simulink model "kalman_estimate_MM"  (R2018b)
settings: Solver=FixedStepAuto  StartTime=0.0  StopTime=500  FixedStep=0.02  RelTol=1e-3
values from neighbouring files (symbols this model uses):
  D = randn(num_output,num_control)    [Com_of_linear_model_calculate.m]    (also in Copy_of_linear_model_calculate.m; D.mat = [0 0 0.00507528406191 0.0236369284061 0.221173094143 0.00198; LINEAR.m = randn(8,1)*10; MM_HKF.m = reshape(out(A_l+B_l+C_l+1:A_l+B_l+C_l+D_l),size_D))
undefined symbols (not defined in the file or in its folder): act_piece, com_piece, piece, sigbuilder_block
libraries: sharedschedule x467, dspsigattribs x44, commchan3 x1
(part 1 of 5)
settings Model: Creator=mmm  LastModifiedBy=mmm

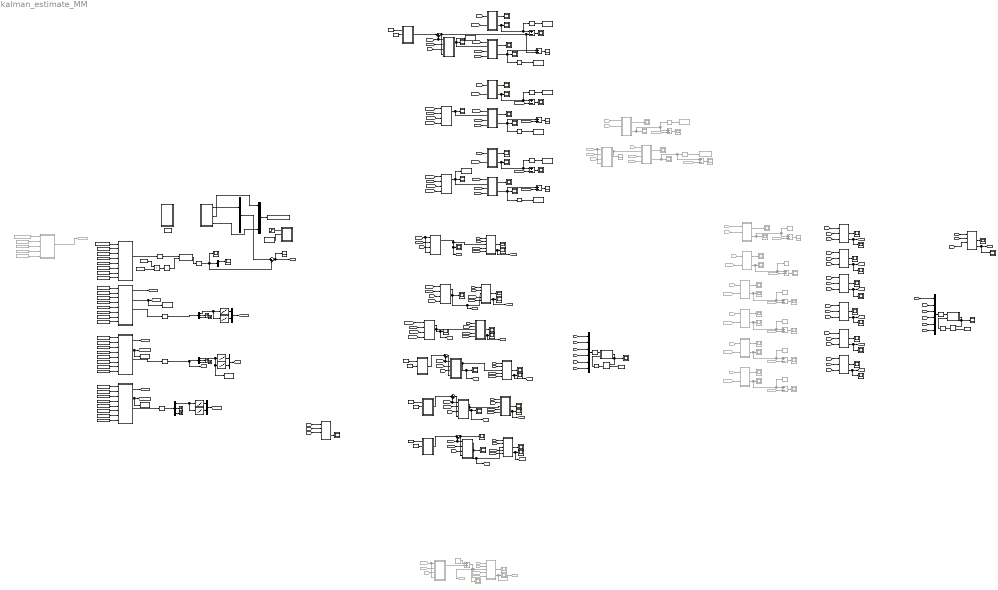
== system kalman_estimate_MM ==
  note: fHPT decrease 3 percent a7
  note: actuator fault a2
  note: T3 fault a5
  note: P21 fault a4
  note: Nh fault a3
  note: boost fault a2
  note: no fault a1
  note: 无故障模式下模型对比
  note: 增压级故障模型对比
  note: 执行机构故障模型对比
  note: 增压级故障模型对比
  1-D Lookup Table1 : Lookup_n-D  NumberOfTableDimensions=1  BreakpointsForDimension1=com_piece.u_stable_(:,1)  Table=com_piece.Nl  InterpMethod=Cubic spline  ExtrapMethod=Cubic spline  InternalRulePriority=Speed  RndMeth=Simplest  InputSameDT=on
  1-D Lookup Table2 : Lookup_n-D  NumberOfTableDimensions=1  BreakpointsForDimension1=piece.u_stable_(:,1)  Table=piece.Nl  InterpMethod=Cubic spline  ExtrapMethod=Cubic spline  InternalRulePriority=Speed  RndMeth=Simplest  InputSameDT=on
  1-D Lookup Table3 : Lookup_n-D  NumberOfTableDimensions=1  BreakpointsForDimension1=piece.u_stable_(:,1)  Table=piece.x_stable_(:,2)  InterpMethod=Cubic spline  ExtrapMethod=Cubic spline  InternalRulePriority=Speed  RndMeth=Simplest  InputSameDT=on
  1-D Lookup Table4 : Lookup_n-D  NumberOfTableDimensions=1  BreakpointsForDimension1=com_piece.u_stable_(:,1)  Table=com_piece.x_stable_(:,2)  InterpMethod=Cubic spline  ExtrapMethod=Cubic spline  InternalRulePriority=Speed  RndMeth=Simplest  InputSameDT=on
  1-D Lookup Table5 : Lookup_n-D  NumberOfTableDimensions=1  BreakpointsForDimension1=act_piece.u_stable_(:,1)  Table=act_piece.Nl  InterpMethod=Cubic spline  ExtrapMethod=Cubic spline  InternalRulePriority=Speed  RndMeth=Simplest  InputSameDT=on
  1-D Lookup Table6 : Lookup_n-D  NumberOfTableDimensions=1  BreakpointsForDimension1=act_piece.u_stable_(:,1)  Table=act_piece.x_stable_(:,2)  InterpMethod=Cubic spline  ExtrapMethod=Cubic spline  InternalRulePriority=Speed  RndMeth=Simplest  InputSameDT=on
  AKF1 : Subsystem
  AKF10 : Subsystem  Commented=on
  AKF12 : Subsystem
  AKF2 : Subsystem
  AKF3 : Subsystem
  AKF4 : Subsystem
  AKF5 : Subsystem
  AKF6 : Subsystem
  AKF7 : Subsystem  Commented=on
  AKF8 : Subsystem
  AKF9 : Subsystem
  AWGN Channel1 : commchan3/AWGN Channel  InputProcessing=Columns as channels (frame based)  seed=51:60  noiseMode=Variance from port  EbNodB=10  EsNodB=10  SNRdB=10  bitsPerSym=1  Ps=1  Tsym=1  variance=[2.55,7.5,0.03,0.03,0.3,0.3,0.15,0.15,0.45,0.45].^2
  Add1 : Sum  Commented=on
  Constant : Constant  Commented=on  Value=[0,0,0,0,0,0,0,0,-0.03,0]  VectorParams1D=off
  Constant{1,4,8,23} (4 alike) : Constant  Value=piece.Ny(:,:,1)
  Constant{10,19,22,24} (4 alike) : Constant  Value=piece.y_index
  Constant{11,25,30,35} (4 alike) : Constant  Value=piece.U_index
  Constant{12,26,31,36} (4 alike) : Constant  Value=piece.x_index
  Constant13 : Constant  Value=[0.051,0.051,0.164,0.164,0.15,0.15,0.23,0.23,0.097,0.097]  VectorParams1D=off
  Constant14 : Constant  Value=0.01
  Constant15 : Constant  Commented=on  Value=piece.HP_index
  Constant16 : Constant  Commented=on  Value=piece.y_index
  Constant17 : Constant  Commented=on  Value=piece.U_index
  Constant18 : Constant  Commented=on  Value=piece.x_index
  Constant{2,27,32,37} (4 alike) : Constant  Value=piece.Nu(:,:,1)
  Constant20 : Constant  Commented=on  Value=piece.mean_design  VectorParams1D=off
  Constant21 : Constant  Value=[0.9,0.01,0.01,0.01,0.01,0.01]  VectorParams1D=off
  Constant{3,28,33,38} (4 alike) : Constant  Value=piece.Nx(:,:,1)
  Constant{9,29,34,39} (4 alike) : Constant  Value=piece.HP_index
  Constant40 : Constant  Value=0
  Constant41 : Constant  Value=[0.9,0.01,0.01,0.01,0.01,0.01]  VectorParams1D=off
  Constant{5..7,42} (4 alike) : Constant  Value=-0.03
  Delay : Delay  DelayLength=1  InitialConditionSource=Input port
      settings: InputPortMap=u0,p4
  Delay1 : Delay  DelayLength=1  InitialConditionSource=Input port
      settings: InputPortMap=u0,p4
  Demux1 : Demux  Outputs=3
  Demux2 : Demux  Outputs=3
  Demux4 : Demux  Outputs=3
  Demux5 : Demux  Outputs=[1,9]
  From{53,71,79,89,92,95,100} (7 alike) : From  Commented=on  GotoTag=y_obem
  From{14,27,39,42,57} (5 alike) : From  Commented=on  GotoTag=y_obem1
  From{21,28,40,47,76} (5 alike) : From  Commented=on  GotoTag=com_x0
  From{26,29,41,46,52,96..97} (7 alike) : From  Commented=on  GotoTag=u
  From{54,69,90..91} (4 alike) : From  Commented=on  GotoTag=x_obem
  From{55..56,72,93..94,99} (6 alike) : From  Commented=on  GotoTag=x0
  From70 : From  Commented=on  GotoTag=y
  Goto31 : Goto  Commented=on  GotoTag=H7
  Goto5 : Goto  Commented=on  GotoTag=y_design
  Goto8 : Goto  Commented=on  GotoTag=f7
  HKF1 : Subsystem
  HKF10 : Subsystem
  HKF11 : Subsystem  Commented=on
  HKF2 : Subsystem
  HKF3 : Subsystem
  HKF4 : Subsystem
  HKF5 : Subsystem
  HKF6 : Subsystem
  HKF7 : Subsystem  Commented=on
  HKF8 : Subsystem
  HKF9 : Subsystem
  MATLAB Function : MATLAB Function  TreatAsAtomicUnit=on
  MATLAB Function1 : MATLAB Function  TreatAsAtomicUnit=on
  MATLAB Function2 : MATLAB Function  TreatAsAtomicUnit=on
  MATLAB Function3 : MATLAB Function  TreatAsAtomicUnit=on
  MATLAB Function4 : MATLAB Function  TreatAsAtomicUnit=on
  MATLAB Function5 : MATLAB Function  TreatAsAtomicUnit=on
  MATLAB Function8 : MATLAB Function  TreatAsAtomicUnit=on
  Math Function : Math  Operator=square  SaturateOnIntegerOverflow=on
  Minus{,3,10..13} (6 alike) : Sum  Inputs=+-
  Minus{1..2,4..9} (8 alike) : Sum  Commented=on  Inputs=+-
  Multiply : Product
  Mux : Mux  Inputs=6
  Mux1 : Mux  Inputs=6
  Mux2 : Mux  Inputs=10
  Mux3 : Mux  Inputs=2
  Mux4 : Mux  Inputs=6
  Mux5 : Mux  Inputs=2
  Mux6 : Mux  Inputs=2
  PIECE kalman : Subsystem
  PIECE kalman1 : Subsystem
  PWL : Subsystem  Commented=on
  Reshape{,4..5,8..9,15..16,19..22} (11 alike) : Reshape  OutputDimensionality=Row vector (2-D)
  Reshape{1,6..7,10..14} (8 alike) : Reshape  Commented=on  OutputDimensionality=Row vector (2-D)
  Reshape{2..3,17..18} (4 alike) : Reshape  OutputDimensionality=Column vector (2-D)
  Scope{1..3,5..6,8..14,16..17,19..21,23..24,26..27,30..32,34..36,38..41,60..88} (60 alike) : Scope
  Scope{4,7,15,18,22,25,28..29,33,37,42..59} (28 alike) : Scope  Commented=on
  Signal Builder : Subsystem  Tag=STV Subsys  LoadFcn=sigbuilder_block('load');  StartFcn=sigbuilder_block('start');  StopFcn=sigbuilder_block('stop');  ClipboardFcn=sigbuilder_block('clipboard');  mask(Sigbuilder block){tuvar=[0:10]}
      mask help: Simulink:masks:SigbuilderBlock_MD
      mask init:
      | if ~strcmp(get_param(bdroot(gcbh),'SimulationStatus'),'stopped') tuvar = sigbuilder_block('maskInit'); end
      settings: CopyFcn=sigbuilder_block('copy');  DeleteFcn=sigbuilder_block('delete');  ModelCloseFcn=sigbuilder_block('modelClose');  PreSaveFcn=sigbuilder_block('preSave');  PauseFcn=sigbuilder_block('pause');  ContinueFcn=sigbuilder_block('continue');  NameChangeFcn=sigbuilder_block('namechange');  OpenFcn=sigbuilder_block('open',[6 30 1428 681 ]);  CloseFcn=sigbuilder_block('close');
      mask Display: plot(0, 0, 100, 100,[2, 2, 32, 32, 2], [68, 8, 8, 68, 68],[32, 2], [38, 38], [32, 19, 2],[53, 60, 44], [32, 17, 17, 2],[16, 16, 31, 31]);txt = getActiveGroup(gcbh);text(2, 100, txt,'verticalAlignment', 'top');
  Signal Builder1 : Subsystem  Tag=STV Subsys  LoadFcn=sigbuilder_block('load');  StartFcn=sigbuilder_block('start');  StopFcn=sigbuilder_block('stop');  ClipboardFcn=sigbuilder_block('clipboard');  mask(Sigbuilder block){tuvar=[0:10]}
      mask help: Simulink:masks:SigbuilderBlock_MD
      mask init:
      | if ~strcmp(get_param(bdroot(gcbh),'SimulationStatus'),'stopped') tuvar = sigbuilder_block('maskInit'); end
      settings: CopyFcn=sigbuilder_block('copy');  DeleteFcn=sigbuilder_block('delete');  ModelCloseFcn=sigbuilder_block('modelClose');  PreSaveFcn=sigbuilder_block('preSave');  PauseFcn=sigbuilder_block('pause');  ContinueFcn=sigbuilder_block('continue');  NameChangeFcn=sigbuilder_block('namechange');  OpenFcn=sigbuilder_block('open',[6 30 1428 681 ]);  CloseFcn=sigbuilder_block('close');
      mask Display: plot(0, 0, 100, 100,[2, 2, 32, 32, 2], [68, 8, 8, 68, 68],[32, 2], [38, 38], [32, 19, 2],[53, 60, 44], [32, 17, 17, 2],[16, 16, 31, 31]);txt = getActiveGroup(gcbh);text(2, 100, txt,'verticalAlignment', 'top');
  Step : Step  Time=100  After=-0.08  SampleTime=0
  Sum{1..5} (5 alike) : Sum  Inputs=|++
  Terminator{1..6} (6 alike) : Terminator
  To Workspace : ToWorkspace  VariableName=fault_vector2  SampleTime=-1
      settings: Save2DSignal=2-D array (concatenate along first dimension)
  To Workspace1 : ToWorkspace  VariableName=y_obem2  SampleTime=-1
      settings: Save2DSignal=2-D array (concatenate along first dimension)
  To Workspace10 : ToWorkspace  VariableName=act_PWL  SampleTime=-1
      settings: Save2DSignal=2-D array (concatenate along first dimension)
  To Workspace11 : ToWorkspace  VariableName=sen3_HP_HKF  SampleTime=-1
      settings: Save2DSignal=2-D array (concatenate along first dimension)
  To Workspace12 : ToWorkspace  VariableName=sen3_PWL  SampleTime=-1
      settings: Save2DSignal=2-D array (concatenate along first dimension)
  To Workspace13 : ToWorkspace  VariableName=act_hp  SampleTime=-1
      settings: Save2DSignal=2-D array (concatenate along first dimension)
  To Workspace14 : ToWorkspace  VariableName=sen3_hp  SampleTime=-1
      settings: Save2DSignal=2-D array (concatenate along first dimension)
  To Workspace2 : ToWorkspace  VariableName=com_HP_HKF  SampleTime=-1
      settings: Save2DSignal=2-D array (concatenate along first dimension)
  To Workspace3 : ToWorkspace  VariableName=u  SaveFormat=Timeseries  SampleTime=-1
  To Workspace4 : ToWorkspace  VariableName=y_obem1  SampleTime=-1
      settings: Save2DSignal=2-D array (concatenate along first dimension)
  To Workspace5 : ToWorkspace  VariableName=com_PWL  SampleTime=-1
      settings: Save2DSignal=2-D array (concatenate along first dimension)
  To Workspace6 : ToWorkspace  Commented=on  VariableName=norm_PWL  SampleTime=-1
      settings: Save2DSignal=2-D array (concatenate along first dimension)
  To Workspace7 : ToWorkspace  Commented=on  VariableName=norm_HP_HKF  SampleTime=-1
      settings: Save2DSignal=2-D array (concatenate along first dimension)
  To Workspace8 : ToWorkspace  VariableName=y_obem  SampleTime=-1
      settings: Save2DSignal=2-D array (concatenate along first dimension)
  To Workspace9 : ToWorkspace  VariableName=act_HP_HKF  SampleTime=-1
      settings: Save2DSignal=2-D array (concatenate along first dimension)
  U1 : FromWorkspace  VariableName=model_test_com  SampleTime=0.02  Interpolate=off  OutputAfterFinalValue=Holding final value
  U2 : FromWorkspace  VariableName=model_test_health  SampleTime=0.02  Interpolate=off  OutputAfterFinalValue=Holding final value
  U3 : FromWorkspace  VariableName=model_test_act  SampleTime=0.02  Interpolate=off  OutputAfterFinalValue=Holding final value
  U4 : FromWorkspace  VariableName=model_test_health  SampleTime=0.02  Interpolate=off  OutputAfterFinalValue=Holding final value
  act_PIECE kalman : Subsystem
  act_PWL : Subsystem  Commented=on
  act_PWL_model : Subsystem
  com_PIECE kalman : Subsystem
  component_PWL : Subsystem  Commented=on
  component_PWL1 : Subsystem
  data_pre : MATLAB Function  TreatAsAtomicUnit=on
  data_pre1 : MATLAB Function  Commented=on  TreatAsAtomicUnit=on
  data_pre2 : MATLAB Function  TreatAsAtomicUnit=on
  data_pre3 : MATLAB Function  TreatAsAtomicUnit=on
  health_PWL : Subsystem  Commented=on
  no. of fault sensor : Constant  Value=8
  no. of fault sensor1 : Constant  Value=3
  no. of fault sensor3 : Constant  Value=2
  no. of fault sensor4 : Constant  Value=3
  no. of fault sensor5 : Constant  Value=8
  real_engine : MATLAB Function  TreatAsAtomicUnit=on
  sen2_PIECE kalman2 : Subsystem
  sen2_PWL : Subsystem  Commented=on
  sen3_PIECE kalman1 : Subsystem
  sen3_PIECE kalman3 : Subsystem
  sen3_PWL : Subsystem  Commented=on
  sen3_PWL-model : Subsystem
  sen8_PIECE kalman : Subsystem
  sen8_PWL : Subsystem  Commented=on
  wires:
  Reshape2/1 -> Demux4/1, [u]
  Demux4/1 -> To Workspace3/1, 1-D Lookup Table3/1, 1-D Lookup Table2/1
  Constant18/1 -> data_pre1/5(x_index)
  Reshape3/1 -> Sum2/2, Demux5/1, Scope10/1
  Constant9/1 -> data_pre/3(HP_index)
  Demux5/1 -> Scope9/1
  data_pre/2(y) -> To Workspace4/1, [y_obem1]
  Reshape/1 -> AWGN Channel1/1
  data_pre1/2(y) -> Goto5/1
  Constant16/1 -> data_pre1/2(y_index)
  Constant17/1 -> data_pre1/4(U_index)
  Constant15/1 -> data_pre1/3(HP_index)
  Constant12/1 -> data_pre/5(x_index)
  Constant11/1 -> data_pre/4(U_index)
  U1/1 -> data_pre/1(row_data)
  1-D Lookup Table2/1 -> Mux5/1
  no. of fault sensor/1 -> MATLAB Function/2(no)
  Constant10/1 -> data_pre/2(y_index)
  Mux5/1 -> [x0]
  1-D Lookup Table3/1 -> Mux5/2
  Constant13/1 -> Multiply/1
  Constant14/1 -> Multiply/2
  AWGN Channel1/1 -> Reshape3/1
  Sum2/1 -> Scope5/1, [y]
  Demux4/3 -> Terminator4/1
  Constant20/1 -> data_pre1/1(row_data)
  Math Function/1 -> AWGN Channel1/2
  Demux4/2 -> Terminator3/1
  Multiply/1 -> Math Function/1
  Constant2/1 -> data_pre/8(Nu)
  Constant1/1 -> data_pre/7(Ny)
  Constant3/1 -> data_pre/6(Nx)
  PIECE kalman/2(Out2) -> Scope12/1
  [u] -> PIECE kalman/1(In1)
  [x0] -> PIECE kalman/3(In3)
  [y] -> PIECE kalman/2(In2)
  data_pre/1(x) -> [x_obem1]
  [y_obem] -> HKF1/5(y_obem)
  [x_obem] -> HKF1/4(x_obem)
  HKF1/2(Out2) -> Scope13/1
  [com_x0] -> HKF1/2(In3)
  [y] -> HKF1/1(In2)
  [x_obem] -> AKF1/2(x_obem)
  [com_x0] -> AKF1/3(x0)
  AKF1/1(hp_est) -> HKF1/3(In4), [H2], Scope1/1
  [y_obem] -> HKF3/5(y_obem)
  [x_obem] -> HKF3/4(x_obem)
  HKF3/2(Out2) -> Scope2/1
  [x0] -> HKF3/2(In3)
  [y] -> HKF3/1(In2)
  [y] -> HKF4/1(In2)
  [x0] -> HKF4/2(In3)
  HKF4/2(Out2) -> Scope3/1
  [x_obem] -> HKF4/4(x_obem)
  [y_obem] -> HKF4/5(y_obem)
  [x_obem] -> AKF3/2(x_obem)
  [x0] -> AKF3/3(x0)
  AKF3/1(hp_est) -> HKF3/3(In4), [H3], Scope6/1
  AKF4/1(hp_est) -> HKF4/3(In4), [H4], Scope8/1
  [x0] -> AKF4/3(x0)
  [x_obem] -> AKF4/2(x_obem)
  Constant5/1 -> MATLAB Function3/1(mag)
  no. of fault sensor3/1 -> MATLAB Function3/2(no)
  no. of fault sensor4/1 -> MATLAB Function4/2(no)
  Constant6/1 -> MATLAB Function4/1(mag)
  Constant7/1 -> MATLAB Function5/1(mag)
  no. of fault sensor5/1 -> MATLAB Function5/2(no)
  [x_obem] -> AKF5/2(x_obem)
  [x0] -> AKF5/3(x0)
  [act_x0] -> AKF6/3(x0)
  [x_obem] -> AKF6/2(x_obem)
  From54/1 -> AKF7/2(x_obem)
  From55/1 -> AKF7/3(x0)
  AKF5/1(hp_est) -> [H5], HKF5/3(In4), Scope11/1
  [y_obem] -> HKF5/5(y_obem)
  [x_obem] -> HKF5/4(x_obem)
  HKF5/2(Out2) -> Scope16/1
  [x0] -> HKF5/2(In3)
  [y] -> HKF5/1(In2)
  [y] -> HKF6/1(In2)
  [x0] -> HKF6/2(In3)
  HKF6/2(Out2) -> Scope17/1
  [x_obem] -> HKF6/4(x_obem)
  [y_obem] -> HKF6/5(y_obem)
  AKF6/1(hp_est) -> [H6], HKF6/3(In4), Scope14/1
  AKF7/1(hp_est) -> Add1/2
  From71/1 -> HKF7/5(y_obem)
  From69/1 -> HKF7/4(x_obem)
  HKF7/2(Out2) -> Scope18/1
  From72/1 -> HKF7/2(In3)
  From70/1 -> HKF7/1(In2)
  [y_obem] -> AKF3/1("y_obem "), Sum3/2
  MATLAB Function3/1(y) -> Sum3/1
  MATLAB Function4/1(y) -> Sum4/1
  [y_obem] -> AKF5/1("y_obem "), Sum5/2
  Sum5/1 -> AKF5/4(y), Scope21/1
  MATLAB Function5/1(y) -> Sum5/1
  [y_obem] -> AKF6/1("y_obem ")
  From53/1 -> AKF7/4(y), AKF7/1("y_obem ")
  [y_obem] -> AKF4/1("y_obem "), Sum4/2
  Sum4/1 -> AKF4/4(y)
  Sum3/1 -> AKF3/4(y)
  [y_obem] -> AKF1/1("y_obem ")
  HKF3/3(Out3) -> [f4], Scope19/1
  HKF4/3(Out3) -> [f5], Scope20/1
  HKF7/3(Out3) -> Goto8/1, Scope22/1
  HKF6/3(Out3) -> [f2], Scope23/1
  HKF5/3(Out3) -> [f6], Scope24/1
  HKF1/3(Out3) -> [f3], Scope26/1
  [f1] -> Mux/1
  Mux/1 -> Reshape4/1
  MATLAB Function8/1(y) -> Delay/1, Scope27/1
  Delay/1 -> Reshape5/1
  Constant21/1 -> Delay/2
  Reshape4/1 -> MATLAB Function8/1(u)
  Reshape5/1 -> MATLAB Function8/2(p0)
  Step/1 -> MATLAB Function/1(mag)
  From56/1 -> PWL/2(In3)
  From46/1 -> PWL/1(In1)
  PWL/1(Out1) -> Scope28/1
  [y_obem] -> AKF8/4(y), AKF8/1("y_obem ")
  [x0] -> AKF8/3(x0)
  [x_obem] -> AKF8/2(x_obem)
  component_PWL1/1(Out1) -> Scope34/1
  component_PWL1/2(Out2) -> Reshape8/1, Minus/1, Scope35/1
  [y_obem1] -> Minus/2
  Minus/1 -> Scope36/1
  1-D Lookup Table4/1 -> Mux3/2
  Mux3/1 -> [com_x0]
  1-D Lookup Table1/1 -> Mux3/1
  [com_x0] -> component_PWL1/2(x0)
  Constant26/1 -> data_pre2/5(x_index)
  Constant25/1 -> data_pre2/4(U_index)
  Constant24/1 -> data_pre2/2(y_index)
  Constant23/1 -> data_pre2/7(Ny)
  Constant29/1 -> data_pre2/3(HP_index)
  Constant28/1 -> data_pre2/6(Nx)
  Constant27/1 -> data_pre2/8(Nu)
  U2/1 -> data_pre2/1(row_data)
  data_pre2/2(y) -> To Workspace8/1, [y_obem]
  data_pre2/1(x) -> [x_obem]
  [y_obem1] -> AKF1/4(y)
  Reshape8/1 -> To Workspace5/1
  [u] -> component_PWL1/1(u)
  HKF10/2(Out2) -> Reshape9/1, Minus3/1, Scope39/1
  Reshape9/1 -> To Workspace2/1
  [y_obem] -> HKF10/4(y_obem)
  [x_obem] -> HKF10/3(x_obem)
  HKF10/1(Out1) -> Scope38/1
  [com_x0] -> HKF10/1(In3)
  [y_obem1] -> AKF9/4(y)
  [y_obem] -> AKF9/1("y_obem ")
  AKF9/1(hp_est) -> HKF10/2(In4), Scope40/1
  [x_obem] -> AKF9/2(x_obem)
  [com_x0] -> AKF9/3(x0)
  [y_obem1] -> Minus3/2
  Minus3/1 -> Scope41/1
  Minus2/1 -> Scope33/1
  Reshape10/1 -> To Workspace6/1
  From79/1 -> Minus2/2
  PWL/2(Out2) -> Minus2/1, Reshape10/1, Scope29/1
  Reshape7/1 -> To Workspace7/1
  From92/1 -> HKF11/4(y_obem)
  From91/1 -> HKF11/3(x_obem)
  HKF11/1(Out1) -> Scope42/1
  From93/1 -> HKF11/1(In3)
  From90/1 -> AKF10/2(x_obem)
  From94/1 -> AKF10/3(x0)
  From89/1 -> AKF10/4(y), AKF10/1("y_obem ")
  AKF10/1(hp_est) -> HKF11/2(In4), Scope37/1
  HKF11/2(Out2) -> Scope43/1, Minus4/1, Reshape7/1
  From95/1 -> Minus4/2
  Minus4/1 -> Scope44/1
  AKF8/1(hp_est) -> HKF9/3(In4), [H1], Scope30/1
  HKF9/3(Out3) -> Scope32/1, [f1]
  [y] -> HKF9/1(In2)
  [x0] -> HKF9/2(In3)
  HKF9/2(Out2) -> Scope31/1
  [x_obem] -> HKF9/4(x_obem)
  [y_obem] -> HKF9/5(y_obem)
  data_pre3/1(x) -> [x_obem2]
  data_pre3/2(y) -> [y_obem2], To Workspace1/1
  U3/1 -> data_pre3/1(row_data)
  Constant32/1 -> data_pre3/8(Nu)
  Constant33/1 -> data_pre3/6(Nx)
  Constant34/1 -> data_pre3/3(HP_index)
  Constant4/1 -> data_pre3/7(Ny)
  Constant22/1 -> data_pre3/2(y_index)
  Constant30/1 -> data_pre3/4(U_index)
  Constant31/1 -> data_pre3/5(x_index)
  [y_obem2] -> AKF6/4(y)
  Constant/1 -> Add1/1
  Add1/1 -> Goto31/1, Scope15/1, HKF7/3(In4)
  Constant38/1 -> real_engine/6(Nx)
  Constant8/1 -> real_engine/7(Ny)
  Constant37/1 -> real_engine/8(Nu)
  Constant19/1 -> real_engine/2(y_index)
  U4/1 -> real_engine/1(row_data)
  Constant35/1 -> real_engine/4(U_index)
  Constant36/1 -> real_engine/5(x_index)
  Constant39/1 -> real_engine/3(HP_index)
  real_engine/2(y) -> Reshape/1
  Mux2/1 -> Sum2/1
  Signal Builder/4(Signal 1) -> Mux1/1
  Signal Builder/6(Signal 6) -> Mux1/6
  Mux1/1 -> To Workspace/1
  sen2_PWL/2(Out2) -> Reshape1/1, Minus1/1, Scope7/1
  From26/1 -> sen2_PWL/1(u)
  Minus1/1 -> Scope25/1
  From14/1 -> Minus1/2
  From21/1 -> sen2_PWL/2(x0)
  sen2_PWL/1(Out1) -> Scope4/1
  Minus5/1 -> Scope45/1
  sen3_PWL/1(Out1) -> Scope46/1
  sen3_PWL/2(Out2) -> Reshape6/1, Minus5/1, Scope47/1
  From27/1 -> Minus5/2
  From28/1 -> sen3_PWL/2(x0)
  From29/1 -> sen3_PWL/1(u)
  From41/1 -> sen8_PWL/1(u)
  From40/1 -> sen8_PWL/2(x0)
  sen8_PWL/2(Out2) -> Reshape11/1, Minus6/1, Scope50/1
  From39/1 -> Minus6/2
  Minus6/1 -> Scope48/1
  sen8_PWL/1(Out1) -> Scope49/1
  component_PWL/2(Out2) -> Reshape12/1, Minus7/1, Scope52/1
  From52/1 -> component_PWL/1(u)
  Minus7/1 -> Scope53/1
  From42/1 -> Minus7/2
  From47/1 -> component_PWL/2(x0)
  component_PWL/1(Out1) -> Scope51/1
  Minus8/1 -> Scope56/1
  From76/1 -> act_PWL/2(x0)
  From57/1 -> Minus8/2
  From96/1 -> act_PWL/1(u)
  act_PWL/1(Out1) -> Scope54/1
  act_PWL/2(Out2) -> Reshape13/1, Minus8/1, Scope55/1
  Minus9/1 -> Scope59/1
  health_PWL/1(Out1) -> Scope57/1
  From100/1 -> Minus9/2
  From97/1 -> health_PWL/1(In1)
  From99/1 -> health_PWL/2(In3)
  health_PWL/2(Out2) -> Minus9/1, Reshape14/1, Scope58/1
  [u] -> PIECE kalman1/1(u)
  [u] -> sen2_PIECE kalman2/1(u)
  [u] -> sen3_PIECE kalman3/1(u)
  [u] -> sen8_PIECE kalman/1(u)
  [u] -> com_PIECE kalman/1(u)
  [u] -> act_PIECE kalman/1(u)
  [y] -> PIECE kalman1/2(y)
  [y] -> sen2_PIECE kalman2/2(y)
  [y] -> sen3_PIECE kalman3/2(y)
  [y] -> sen8_PIECE kalman/2(y)
  [y] -> com_PIECE kalman/2(y)
  [y] -> act_PIECE kalman/2(y)
  Constant41/1 -> Delay1/2
  Reshape15/1 -> MATLAB Function1/1(u)
  Reshape16/1 -> MATLAB Function1/2(p0)
  Mux4/1 -> Reshape15/1
  MATLAB Function1/1(y) -> Delay1/1, Scope60/1
  [ff1] -> Mux4/1
  Delay1/1 -> Reshape16/1
  PIECE kalman1/3(Out3) -> Scope61/1, [ff11]
  sen2_PIECE kalman2/3(Out3) -> Scope62/1, [ff4]
  sen3_PIECE kalman3/3(Out3) -> Scope63/1, [ff5]
  sen8_PIECE kalman/3(Out3) -> Scope64/1, [ff6]
  com_PIECE kalman/3(Out3) -> Scope65/1, [ff3]
  act_PIECE kalman/3(Out3) -> Scope66/1, [ff2]
  [x0] -> PIECE kalman1/3(x0)
  [x0] -> sen2_PIECE kalman2/3(x0)
  [x0] -> sen3_PIECE kalman3/3(x0)
  [x0] -> sen8_PIECE kalman/3(x0)
  [x0] -> com_PIECE kalman/3(x0)
  [x0] -> act_PIECE kalman/3(x0)
  PIECE kalman1/2(Out2) -> Scope67/1
  sen2_PIECE kalman2/2(Out2) -> Scope68/1
  sen3_PIECE kalman3/2(Out2) -> Scope69/1
  sen8_PIECE kalman/2(Out2) -> Scope70/1
  com_PIECE kalman/2(Out2) -> Scope71/1
  act_PIECE kalman/2(Out2) -> Scope72/1
  sen3_PIECE kalman1/2(Out2) -> Scope74/1
  [x0] -> sen3_PIECE kalman1/3(x0)
  sen3_PIECE kalman1/3(Out3) -> [ff1], Scope73/1
  [y] -> sen3_PIECE kalman1/2(y)
  [u] -> sen3_PIECE kalman1/1(u)
  [f2] -> Mux/2
  [f3] -> Mux/3
  [f4] -> Mux/4
  [f5] -> Mux/5
  [f6] -> Mux/6
  [ff2] -> Mux4/2
  [ff3] -> Mux4/3
  [ff4] -> Mux4/4
  [ff5] -> Mux4/5
  [ff6] -> Mux4/6
  1-D Lookup Table5/1 -> Mux6/1
  Mux6/1 -> [act_x0]
  1-D Lookup Table6/1 -> Mux6/2
  Signal Builder/1(Signal 2) -> Mux2/3
  data_pre3/3(U) -> Reshape17/1
  Demux1/2 -> Terminator1/1
  Demux1/3 -> Terminator2/1
  Reshape17/1 -> Demux1/1
  Demux1/1 -> 1-D Lookup Table6/1, 1-D Lookup Table5/1
  Demux2/2 -> Terminator5/1
  Demux2/3 -> Terminator6/1
  Reshape18/1 -> Demux2/1
  data_pre2/3(U) -> Reshape2/1
  Demux2/1 -> 1-D Lookup Table4/1, 1-D Lookup Table1/1
  data_pre/3(U) -> Reshape18/1
  Minus11/1 -> Scope81/1
  [y_obem2] -> Minus11/2
  [act_x0] -> AKF2/3(x0)
  [x_obem] -> AKF2/2(x_obem)
  AKF2/1(hp_est) -> To Workspace13/1, Scope80/1, HKF2/2(In4)
  [y_obem] -> AKF2/1("y_obem ")
  [y_obem2] -> AKF2/4(y)
  [act_x0] -> HKF2/1(In3)
  HKF2/1(Out1) -> Scope78/1
  [x_obem] -> HKF2/3(x_obem)
  [y_obem] -> HKF2/4(y_obem)
  Reshape20/1 -> To Workspace9/1
  HKF2/2(Out2) -> Scope79/1, Minus11/1, Reshape20/1
  [u] -> act_PWL_model/1(u)
  Reshape19/1 -> To Workspace10/1
  [act_x0] -> act_PWL_model/2(x0)
  Minus10/1 -> Scope77/1
  [y_obem2] -> Minus10/2
  act_PWL_model/2(Out2) -> Scope76/1, Minus10/1, Reshape19/1
  act_PWL_model/1(Out1) -> Scope75/1
  HKF8/1(Out1) -> Scope85/1
  Sum1/1 -> Minus13/2, Minus12/2, AKF12/4(y)
  [x_obem] -> HKF8/3(x_obem)
  Minus12/1 -> Scope84/1
  Minus13/1 -> Scope88/1
  [x0] -> HKF8/1(In3)
  [y_obem] -> HKF8/4(y_obem)
  Reshape22/1 -> To Workspace11/1
  [x0] -> sen3_PWL-model/2(x0)
  Reshape21/1 -> To Workspace12/1
  HKF8/2(Out2) -> Reshape22/1, Minus13/1, Scope86/1
  [u] -> sen3_PWL-model/1(u)
  sen3_PWL-model/1(Out1) -> Scope82/1
  sen3_PWL-model/2(Out2) -> Reshape21/1, Minus12/1, Scope83/1
  Constant42/1 -> MATLAB Function2/1(mag)
  no. of fault sensor1/1 -> MATLAB Function2/2(no)
  [y_obem] -> Sum1/2, AKF12/1("y_obem ")
  MATLAB Function2/1(y) -> Sum1/1
  [x_obem] -> AKF12/2(x_obem)
  [x0] -> AKF12/3(x0)
  AKF12/1(hp_est) -> To Workspace14/1, HKF8/2(In4), Scope87/1

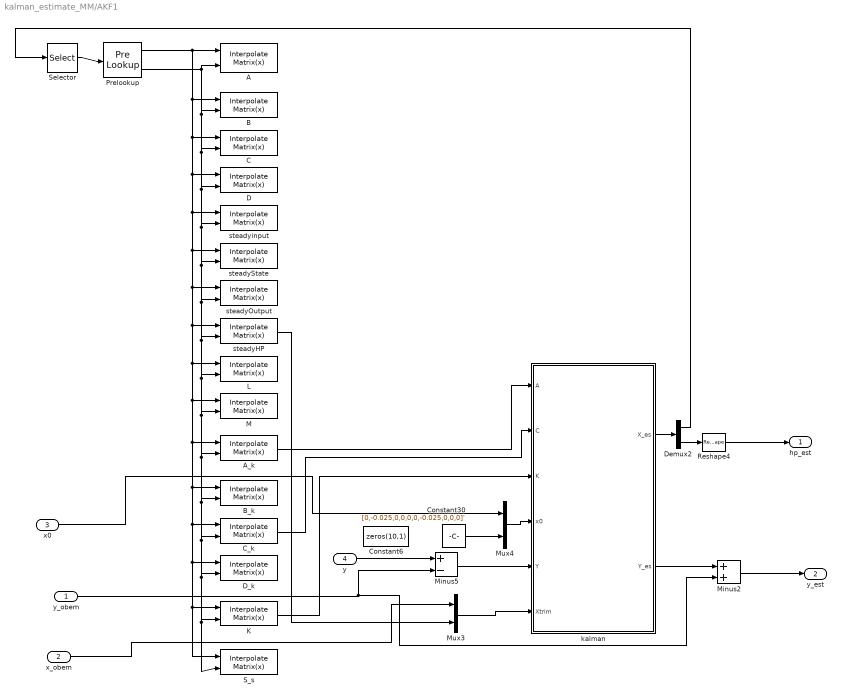
== system kalman_estimate_MM/AKF1 ==
  "y_obem " : Inport
  x_obem : Inport  Port=2
  x0 : Inport  Port=3
  y : Inport  Port=4
  A : sharedschedule/Interpolate Matrix(x)   matrix=piece.A  aMode=aMode
      settings: SourceProductName=Aerospace Blockset  SourceProductBaseCode=AE
  A_k : sharedschedule/Interpolate Matrix(x)   matrix=piece.A_k  aMode=aMode
      settings: SourceProductName=Aerospace Blockset  SourceProductBaseCode=AE
  B : sharedschedule/Interpolate Matrix(x)   matrix=piece.B  aMode=aMode
      settings: SourceProductName=Aerospace Blockset  SourceProductBaseCode=AE
  B_k : sharedschedule/Interpolate Matrix(x)   matrix=piece.B_k  aMode=aMode
      settings: SourceProductName=Aerospace Blockset  SourceProductBaseCode=AE
  C : sharedschedule/Interpolate Matrix(x)   matrix=piece.C  aMode=aMode
      settings: SourceProductName=Aerospace Blockset  SourceProductBaseCode=AE
  C_k : sharedschedule/Interpolate Matrix(x)   matrix=piece.C_k  aMode=aMode
      settings: SourceProductName=Aerospace Blockset  SourceProductBaseCode=AE
  Constant30 : Constant  Value=[0,-0.025,0,0,0,0,-0.025,0,0,0]'  VectorParams1D=off
  Constant6 : Constant  Value=zeros(10,1)  VectorParams1D=off
  D : sharedschedule/Interpolate Matrix(x)   matrix=piece.D  aMode=aMode
      settings: SourceProductName=Aerospace Blockset  SourceProductBaseCode=AE
  D_k : sharedschedule/Interpolate Matrix(x)   matrix=piece.D_k  aMode=aMode
      settings: SourceProductName=Aerospace Blockset  SourceProductBaseCode=AE
  Demux2 : Demux  Outputs=[2,10]
  K : sharedschedule/Interpolate Matrix(x)   matrix=piece.K  aMode=aMode
      settings: SourceProductName=Aerospace Blockset  SourceProductBaseCode=AE
  L : sharedschedule/Interpolate Matrix(x)   matrix=piece.L  aMode=aMode
      settings: SourceProductName=Aerospace Blockset  SourceProductBaseCode=AE
  M : sharedschedule/Interpolate Matrix(x)   matrix=piece.M  aMode=aMode
      settings: SourceProductName=Aerospace Blockset  SourceProductBaseCode=AE
  Minus2 : Sum
  Minus5 : Sum  Inputs=+-
  Mux3 : Mux  Inputs=2
  Mux4 : Mux  Inputs=2
  Prelookup : PreLookup  BreakpointsData=piece.Nl  BreakpointObject=Nl  ExtrapMethod=Linear  UseLastBreakpoint=on  DiagnosticForOutOfRangeInput=Warning
  Reshape4 : Reshape  OutputDimensionality=Row vector (2-D)
  S_s : sharedschedule/Interpolate Matrix(x)   matrix=piece.K_s  aMode=aMode
      settings: SourceProductName=Aerospace Blockset  SourceProductBaseCode=AE
  Selector : Selector  InputPortWidth=2  IndexOptions=Index vector (dialog)  Indices=[1]  OutputSizes=1
  "kalman " : Subsystem
  steadyHP : sharedschedule/Interpolate Matrix(x)   matrix=piece.steadyHP  aMode=aMode
      settings: SourceProductName=Aerospace Blockset  SourceProductBaseCode=AE
  steadyOutput : sharedschedule/Interpolate Matrix(x)   matrix=piece.steadyOutput  aMode=aMode
      settings: SourceProductName=Aerospace Blockset  SourceProductBaseCode=AE
  steadyState : sharedschedule/Interpolate Matrix(x)   matrix=piece.steadyState  aMode=aMode
      settings: SourceProductName=Aerospace Blockset  SourceProductBaseCode=AE
  steadyinput : sharedschedule/Interpolate Matrix(x)   matrix=piece.steadyInput  aMode=aMode
      settings: SourceProductName=Aerospace Blockset  SourceProductBaseCode=AE
  hp_est : Outport
  y_est : Outport  Port=2
  wires:
  Reshape4/1 -> hp_est/1
  Prelookup/2 -> A/2, S_s/2, K/2, D_k/2, C_k/2, B_k/2, A_k/2, M/2, L/2, steadyHP/2, steadyOutput/2, steadyState/2, steadyinput/2, D/2, C/2, B/2
  Prelookup/1 -> S_s/1, K/1, D_k/1, C_k/1, B_k/1, A_k/1, M/1, L/1, steadyHP/1, steadyOutput/1, steadyState/1, steadyinput/1, D/1, C/1, B/1, A/1
  K/1 -> "kalman "/3(K)
  Selector/1 -> Prelookup/1
  x0/1 -> Mux4/1
  A_k/1 -> "kalman "/1(A)
  "kalman "/1(X_es) -> Demux2/1
  Demux2/1 -> Selector/1
  "kalman "/2(Y_es) -> Minus2/1
  Mux3/1 -> "kalman "/6(Xtrim)
  y/1 -> Minus5/1
  Minus5/1 -> "kalman "/5(Y)
  Demux2/2 -> Reshape4/1
  C_k/1 -> "kalman "/2(C)
  "y_obem "/1 -> Minus2/2, Minus5/2
  Mux4/1 -> "kalman "/4(x0)
  steadyHP/1 -> Mux3/2
  Minus2/1 -> y_est/1
  x_obem/1 -> Mux3/1
  Constant30/1 -> Mux4/2

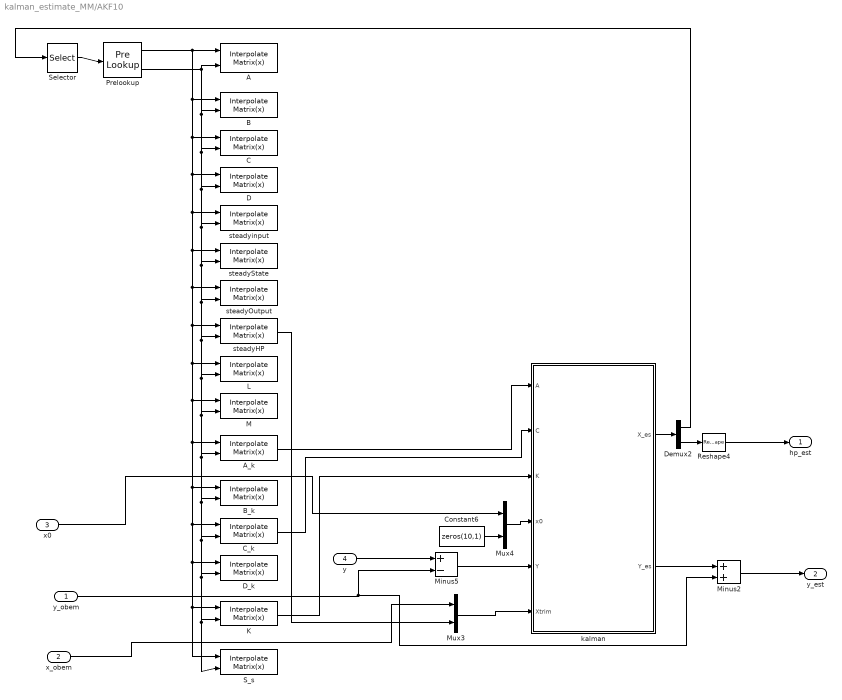
== system kalman_estimate_MM/AKF10 ==
  "y_obem " : Inport
  x_obem : Inport  Port=2
  x0 : Inport  Port=3
  y : Inport  Port=4
  A : sharedschedule/Interpolate Matrix(x)   matrix=piece.A  aMode=aMode
      settings: SourceProductName=Aerospace Blockset  SourceProductBaseCode=AE
  A_k : sharedschedule/Interpolate Matrix(x)   matrix=piece.A_k  aMode=aMode
      settings: SourceProductName=Aerospace Blockset  SourceProductBaseCode=AE
  B : sharedschedule/Interpolate Matrix(x)   matrix=piece.B  aMode=aMode
      settings: SourceProductName=Aerospace Blockset  SourceProductBaseCode=AE
  B_k : sharedschedule/Interpolate Matrix(x)   matrix=piece.B_k  aMode=aMode
      settings: SourceProductName=Aerospace Blockset  SourceProductBaseCode=AE
  C : sharedschedule/Interpolate Matrix(x)   matrix=piece.C  aMode=aMode
      settings: SourceProductName=Aerospace Blockset  SourceProductBaseCode=AE
  C_k : sharedschedule/Interpolate Matrix(x)   matrix=piece.C_k  aMode=aMode
      settings: SourceProductName=Aerospace Blockset  SourceProductBaseCode=AE
  Constant6 : Constant  Value=zeros(10,1)  VectorParams1D=off
  D : sharedschedule/Interpolate Matrix(x)   matrix=piece.D  aMode=aMode
      settings: SourceProductName=Aerospace Blockset  SourceProductBaseCode=AE
  D_k : sharedschedule/Interpolate Matrix(x)   matrix=piece.D_k  aMode=aMode
      settings: SourceProductName=Aerospace Blockset  SourceProductBaseCode=AE
  Demux2 : Demux  Outputs=[2,10]
  K : sharedschedule/Interpolate Matrix(x)   matrix=piece.K  aMode=aMode
      settings: SourceProductName=Aerospace Blockset  SourceProductBaseCode=AE
  L : sharedschedule/Interpolate Matrix(x)   matrix=piece.L  aMode=aMode
      settings: SourceProductName=Aerospace Blockset  SourceProductBaseCode=AE
  M : sharedschedule/Interpolate Matrix(x)   matrix=piece.M  aMode=aMode
      settings: SourceProductName=Aerospace Blockset  SourceProductBaseCode=AE
  Minus2 : Sum
  Minus5 : Sum  Inputs=+-
  Mux3 : Mux  Inputs=2
  Mux4 : Mux  Inputs=2
  Prelookup : PreLookup  BreakpointsData=piece.Nl  BreakpointObject=Nl  ExtrapMethod=Linear  UseLastBreakpoint=on  DiagnosticForOutOfRangeInput=Warning
  Reshape4 : Reshape  OutputDimensionality=Row vector (2-D)
  S_s : sharedschedule/Interpolate Matrix(x)   matrix=piece.K_s  aMode=aMode
      settings: SourceProductName=Aerospace Blockset  SourceProductBaseCode=AE
  Selector : Selector  InputPortWidth=2  IndexOptions=Index vector (dialog)  Indices=[1]  OutputSizes=1
  "kalman " : Subsystem
  steadyHP : sharedschedule/Interpolate Matrix(x)   matrix=piece.steadyHP  aMode=aMode
      settings: SourceProductName=Aerospace Blockset  SourceProductBaseCode=AE
  steadyOutput : sharedschedule/Interpolate Matrix(x)   matrix=piece.steadyOutput  aMode=aMode
      settings: SourceProductName=Aerospace Blockset  SourceProductBaseCode=AE
  steadyState : sharedschedule/Interpolate Matrix(x)   matrix=piece.steadyState  aMode=aMode
      settings: SourceProductName=Aerospace Blockset  SourceProductBaseCode=AE
  steadyinput : sharedschedule/Interpolate Matrix(x)   matrix=piece.steadyInput  aMode=aMode
      settings: SourceProductName=Aerospace Blockset  SourceProductBaseCode=AE
  hp_est : Outport
  y_est : Outport  Port=2
  wires:
  Reshape4/1 -> hp_est/1
  Prelookup/2 -> A/2, S_s/2, K/2, D_k/2, C_k/2, B_k/2, A_k/2, M/2, L/2, steadyHP/2, steadyOutput/2, steadyState/2, steadyinput/2, D/2, C/2, B/2
  Prelookup/1 -> S_s/1, K/1, D_k/1, C_k/1, B_k/1, A_k/1, M/1, L/1, steadyHP/1, steadyOutput/1, steadyState/1, steadyinput/1, D/1, C/1, B/1, A/1
  K/1 -> "kalman "/3(K)
  Selector/1 -> Prelookup/1
  x0/1 -> Mux4/1
  A_k/1 -> "kalman "/1(A)
  "kalman "/1(X_es) -> Demux2/1
  Demux2/1 -> Selector/1
  "kalman "/2(Y_es) -> Minus2/1
  Mux3/1 -> "kalman "/6(Xtrim)
  y/1 -> Minus5/1
  Minus5/1 -> "kalman "/5(Y)
  Demux2/2 -> Reshape4/1
  C_k/1 -> "kalman "/2(C)
  "y_obem "/1 -> Minus2/2, Minus5/2
  Mux4/1 -> "kalman "/4(x0)
  Constant6/1 -> Mux4/2
  steadyHP/1 -> Mux3/2
  Minus2/1 -> y_est/1
  x_obem/1 -> Mux3/1

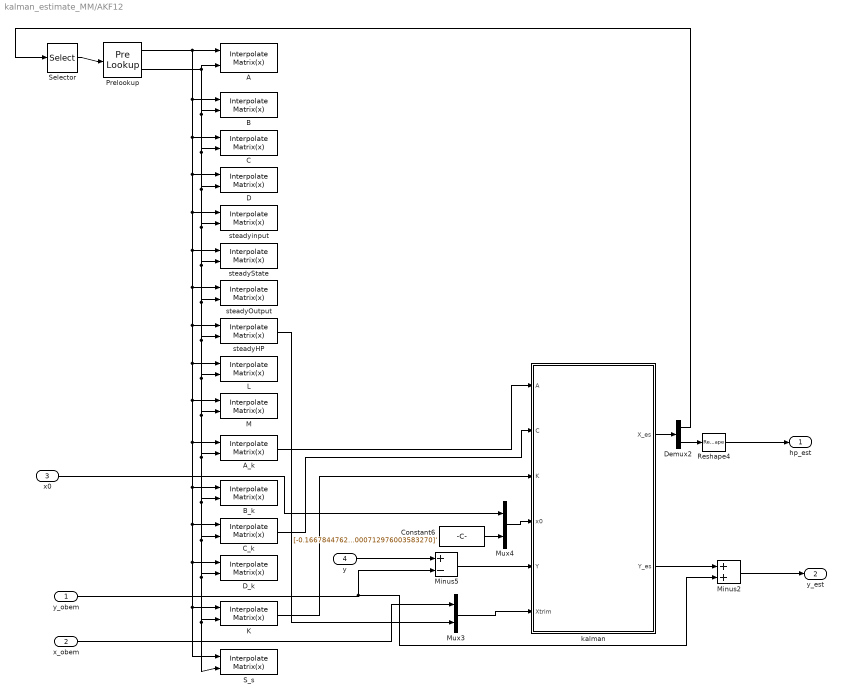
== system kalman_estimate_MM/AKF12 ==
  "y_obem " : Inport
  x_obem : Inport  Port=2
  x0 : Inport  Port=3
  y : Inport  Port=4
  A : sharedschedule/Interpolate Matrix(x)   matrix=piece.A  aMode=aMode
      settings: SourceProductName=Aerospace Blockset  SourceProductBaseCode=AE
  A_k : sharedschedule/Interpolate Matrix(x)   matrix=piece.A_k  aMode=aMode
      settings: SourceProductName=Aerospace Blockset  SourceProductBaseCode=AE
  B : sharedschedule/Interpolate Matrix(x)   matrix=piece.B  aMode=aMode
      settings: SourceProductName=Aerospace Blockset  SourceProductBaseCode=AE
  B_k : sharedschedule/Interpolate Matrix(x)   matrix=piece.B_k  aMode=aMode
      settings: SourceProductName=Aerospace Blockset  SourceProductBaseCode=AE
  C : sharedschedule/Interpolate Matrix(x)   matrix=piece.C  aMode=aMode
      settings: SourceProductName=Aerospace Blockset  SourceProductBaseCode=AE
  C_k : sharedschedule/Interpolate Matrix(x)   matrix=piece.C_k  aMode=aMode
      settings: SourceProductName=Aerospace Blockset  SourceProductBaseCode=AE
  Constant6 : Constant  Value="[-0.166784476259486\t0.0569881075326451\t0.00125702690401568\t-2.45080075419044e-05\t-0.156069579016969\t-0.0654642347822966\t0.0370528098061379\t0.00422624294587915\t7.13880524967784e-05\t0.000712976003583270]'"  VectorParams1D=off
  D : sharedschedule/Interpolate Matrix(x)   matrix=piece.D  aMode=aMode
      settings: SourceProductName=Aerospace Blockset  SourceProductBaseCode=AE
  D_k : sharedschedule/Interpolate Matrix(x)   matrix=piece.D_k  aMode=aMode
      settings: SourceProductName=Aerospace Blockset  SourceProductBaseCode=AE
  Demux2 : Demux  Outputs=[2,10]
  K : sharedschedule/Interpolate Matrix(x)   matrix=piece.K  aMode=aMode
      settings: SourceProductName=Aerospace Blockset  SourceProductBaseCode=AE
  L : sharedschedule/Interpolate Matrix(x)   matrix=piece.L  aMode=aMode
      settings: SourceProductName=Aerospace Blockset  SourceProductBaseCode=AE
  M : sharedschedule/Interpolate Matrix(x)   matrix=piece.M  aMode=aMode
      settings: SourceProductName=Aerospace Blockset  SourceProductBaseCode=AE
  Minus2 : Sum
  Minus5 : Sum  Inputs=+-
  Mux3 : Mux  Inputs=2
  Mux4 : Mux  Inputs=2
  Prelookup : PreLookup  BreakpointsData=piece.Nl  BreakpointObject=Nl  ExtrapMethod=Linear  UseLastBreakpoint=on  DiagnosticForOutOfRangeInput=Warning
  Reshape4 : Reshape  OutputDimensionality=Row vector (2-D)
  S_s : sharedschedule/Interpolate Matrix(x)   matrix=piece.K_s  aMode=aMode
      settings: SourceProductName=Aerospace Blockset  SourceProductBaseCode=AE
  Selector : Selector  InputPortWidth=2  IndexOptions=Index vector (dialog)  Indices=[1]  OutputSizes=1
  "kalman " : Subsystem
  steadyHP : sharedschedule/Interpolate Matrix(x)   matrix=piece.steadyHP  aMode=aMode
      settings: SourceProductName=Aerospace Blockset  SourceProductBaseCode=AE
  steadyOutput : sharedschedule/Interpolate Matrix(x)   matrix=piece.steadyOutput  aMode=aMode
      settings: SourceProductName=Aerospace Blockset  SourceProductBaseCode=AE
  steadyState : sharedschedule/Interpolate Matrix(x)   matrix=piece.steadyState  aMode=aMode
      settings: SourceProductName=Aerospace Blockset  SourceProductBaseCode=AE
  steadyinput : sharedschedule/Interpolate Matrix(x)   matrix=piece.steadyInput  aMode=aMode
      settings: SourceProductName=Aerospace Blockset  SourceProductBaseCode=AE
  hp_est : Outport
  y_est : Outport  Port=2
  wires:
  x_obem/1 -> Mux3/1
  Minus2/1 -> y_est/1
  steadyHP/1 -> Mux3/2
  Constant6/1 -> Mux4/2
  Mux4/1 -> "kalman "/4(x0)
  "y_obem "/1 -> Minus5/2, Minus2/2
  C_k/1 -> "kalman "/2(C)
  Demux2/2 -> Reshape4/1
  Minus5/1 -> "kalman "/5(Y)
  y/1 -> Minus5/1
  Mux3/1 -> "kalman "/6(Xtrim)
  "kalman "/2(Y_es) -> Minus2/1
  Demux2/1 -> Selector/1
  "kalman "/1(X_es) -> Demux2/1
  A_k/1 -> "kalman "/1(A)
  x0/1 -> Mux4/1
  Selector/1 -> Prelookup/1
  K/1 -> "kalman "/3(K)
  Prelookup/1 -> A/1, B/1, C/1, D/1, steadyinput/1, steadyState/1, steadyOutput/1, steadyHP/1, L/1, M/1, A_k/1, B_k/1, C_k/1, D_k/1, K/1, S_s/1
  Prelookup/2 -> B/2, C/2, D/2, steadyinput/2, steadyState/2, steadyOutput/2, steadyHP/2, L/2, M/2, A_k/2, B_k/2, C_k/2, D_k/2, K/2, S_s/2, A/2
  Reshape4/1 -> hp_est/1

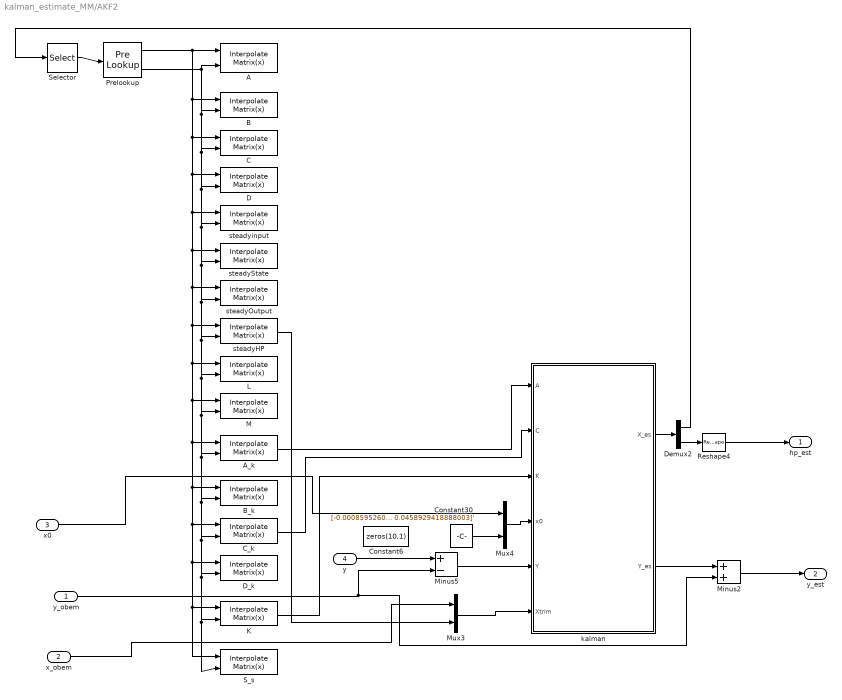
== system kalman_estimate_MM/AKF2 ==
  "y_obem " : Inport
  x_obem : Inport  Port=2
  x0 : Inport  Port=3
  y : Inport  Port=4
  A : sharedschedule/Interpolate Matrix(x)   matrix=piece.A  aMode=aMode
      settings: SourceProductName=Aerospace Blockset  SourceProductBaseCode=AE
  A_k : sharedschedule/Interpolate Matrix(x)   matrix=piece.A_k  aMode=aMode
      settings: SourceProductName=Aerospace Blockset  SourceProductBaseCode=AE
  B : sharedschedule/Interpolate Matrix(x)   matrix=piece.B  aMode=aMode
      settings: SourceProductName=Aerospace Blockset  SourceProductBaseCode=AE
  B_k : sharedschedule/Interpolate Matrix(x)   matrix=piece.B_k  aMode=aMode
      settings: SourceProductName=Aerospace Blockset  SourceProductBaseCode=AE
  C : sharedschedule/Interpolate Matrix(x)   matrix=piece.C  aMode=aMode
      settings: SourceProductName=Aerospace Blockset  SourceProductBaseCode=AE
  C_k : sharedschedule/Interpolate Matrix(x)   matrix=piece.C_k  aMode=aMode
      settings: SourceProductName=Aerospace Blockset  SourceProductBaseCode=AE
  Constant30 : Constant  Value="[-0.000859526083722872\t-0.0176831317558311\t-0.00203166203425789\t0.00151414469013444\t-0.0221737327589031\t0.00177980317723996\t0.0184269320931292\t0.0303443103995220\t0.0477278519877635\t0.0458929418888003]'"  VectorParams1D=off
  Constant6 : Constant  Value=zeros(10,1)  VectorParams1D=off
  D : sharedschedule/Interpolate Matrix(x)   matrix=piece.D  aMode=aMode
      settings: SourceProductName=Aerospace Blockset  SourceProductBaseCode=AE
  D_k : sharedschedule/Interpolate Matrix(x)   matrix=piece.D_k  aMode=aMode
      settings: SourceProductName=Aerospace Blockset  SourceProductBaseCode=AE
  Demux2 : Demux  Outputs=[2,10]
  K : sharedschedule/Interpolate Matrix(x)   matrix=piece.K  aMode=aMode
      settings: SourceProductName=Aerospace Blockset  SourceProductBaseCode=AE
  L : sharedschedule/Interpolate Matrix(x)   matrix=piece.L  aMode=aMode
      settings: SourceProductName=Aerospace Blockset  SourceProductBaseCode=AE
  M : sharedschedule/Interpolate Matrix(x)   matrix=piece.M  aMode=aMode
      settings: SourceProductName=Aerospace Blockset  SourceProductBaseCode=AE
  Minus2 : Sum
  Minus5 : Sum  Inputs=+-
  Mux3 : Mux  Inputs=2
  Mux4 : Mux  Inputs=2
  Prelookup : PreLookup  BreakpointsData=piece.Nl  BreakpointObject=Nl  ExtrapMethod=Linear  UseLastBreakpoint=on  DiagnosticForOutOfRangeInput=Warning
  Reshape4 : Reshape  OutputDimensionality=Row vector (2-D)
  S_s : sharedschedule/Interpolate Matrix(x)   matrix=piece.K_s  aMode=aMode
      settings: SourceProductName=Aerospace Blockset  SourceProductBaseCode=AE
  Selector : Selector  InputPortWidth=2  IndexOptions=Index vector (dialog)  Indices=[1]  OutputSizes=1
  "kalman " : Subsystem
  steadyHP : sharedschedule/Interpolate Matrix(x)   matrix=piece.steadyHP  aMode=aMode
      settings: SourceProductName=Aerospace Blockset  SourceProductBaseCode=AE
  steadyOutput : sharedschedule/Interpolate Matrix(x)   matrix=piece.steadyOutput  aMode=aMode
      settings: SourceProductName=Aerospace Blockset  SourceProductBaseCode=AE
  steadyState : sharedschedule/Interpolate Matrix(x)   matrix=piece.steadyState  aMode=aMode
      settings: SourceProductName=Aerospace Blockset  SourceProductBaseCode=AE
  steadyinput : sharedschedule/Interpolate Matrix(x)   matrix=piece.steadyInput  aMode=aMode
      settings: SourceProductName=Aerospace Blockset  SourceProductBaseCode=AE
  hp_est : Outport
  y_est : Outport  Port=2
  wires:
  Constant30/1 -> Mux4/2
  x_obem/1 -> Mux3/1
  Minus2/1 -> y_est/1
  steadyHP/1 -> Mux3/2
  Mux4/1 -> "kalman "/4(x0)
  "y_obem "/1 -> Minus5/2, Minus2/2
  C_k/1 -> "kalman "/2(C)
  Demux2/2 -> Reshape4/1
  Minus5/1 -> "kalman "/5(Y)
  y/1 -> Minus5/1
  Mux3/1 -> "kalman "/6(Xtrim)
  "kalman "/2(Y_es) -> Minus2/1
  Demux2/1 -> Selector/1
  "kalman "/1(X_es) -> Demux2/1
  A_k/1 -> "kalman "/1(A)
  x0/1 -> Mux4/1
  Selector/1 -> Prelookup/1
  K/1 -> "kalman "/3(K)
  Prelookup/1 -> A/1, B/1, C/1, D/1, steadyinput/1, steadyState/1, steadyOutput/1, steadyHP/1, L/1, M/1, A_k/1, B_k/1, C_k/1, D_k/1, K/1, S_s/1
  Prelookup/2 -> B/2, C/2, D/2, steadyinput/2, steadyState/2, steadyOutput/2, steadyHP/2, L/2, M/2, A_k/2, B_k/2, C_k/2, D_k/2, K/2, S_s/2, A/2
  Reshape4/1 -> hp_est/1

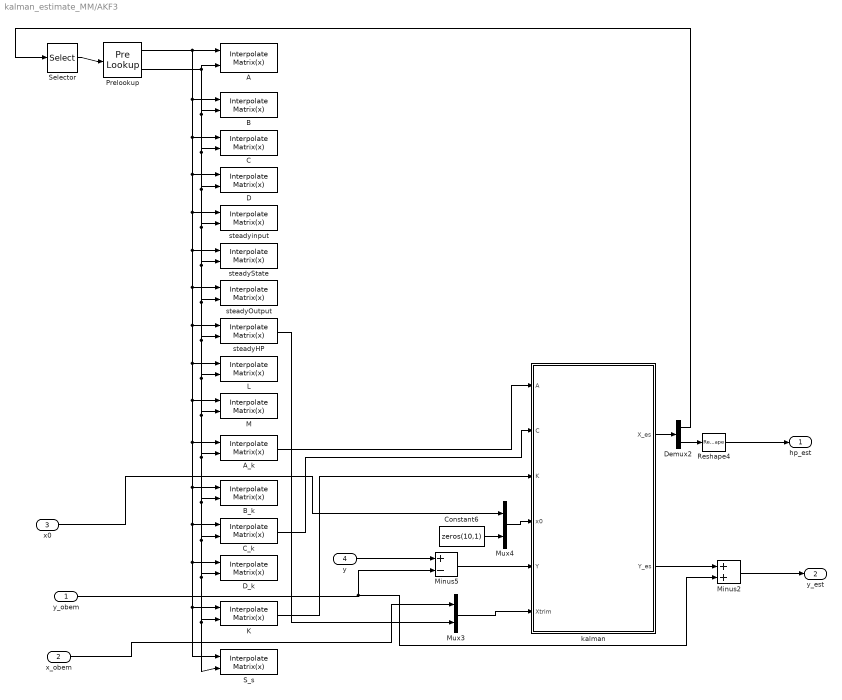
== system kalman_estimate_MM/AKF3 ==
  "y_obem " : Inport
  x_obem : Inport  Port=2
  x0 : Inport  Port=3
  y : Inport  Port=4
  A : sharedschedule/Interpolate Matrix(x)   matrix=piece.A  aMode=aMode
      settings: SourceProductName=Aerospace Blockset  SourceProductBaseCode=AE
  A_k : sharedschedule/Interpolate Matrix(x)   matrix=piece.A_k  aMode=aMode
      settings: SourceProductName=Aerospace Blockset  SourceProductBaseCode=AE
  B : sharedschedule/Interpolate Matrix(x)   matrix=piece.B  aMode=aMode
      settings: SourceProductName=Aerospace Blockset  SourceProductBaseCode=AE
  B_k : sharedschedule/Interpolate Matrix(x)   matrix=piece.B_k  aMode=aMode
      settings: SourceProductName=Aerospace Blockset  SourceProductBaseCode=AE
  C : sharedschedule/Interpolate Matrix(x)   matrix=piece.C  aMode=aMode
      settings: SourceProductName=Aerospace Blockset  SourceProductBaseCode=AE
  C_k : sharedschedule/Interpolate Matrix(x)   matrix=piece.C_k  aMode=aMode
      settings: SourceProductName=Aerospace Blockset  SourceProductBaseCode=AE
  Constant6 : Constant  Value=zeros(10,1)  VectorParams1D=off
  D : sharedschedule/Interpolate Matrix(x)   matrix=piece.D  aMode=aMode
      settings: SourceProductName=Aerospace Blockset  SourceProductBaseCode=AE
  D_k : sharedschedule/Interpolate Matrix(x)   matrix=piece.D_k  aMode=aMode
      settings: SourceProductName=Aerospace Blockset  SourceProductBaseCode=AE
  Demux2 : Demux  Outputs=[2,10]
  K : sharedschedule/Interpolate Matrix(x)   matrix=piece.K  aMode=aMode
      settings: SourceProductName=Aerospace Blockset  SourceProductBaseCode=AE
  L : sharedschedule/Interpolate Matrix(x)   matrix=piece.L  aMode=aMode
      settings: SourceProductName=Aerospace Blockset  SourceProductBaseCode=AE
  M : sharedschedule/Interpolate Matrix(x)   matrix=piece.M  aMode=aMode
      settings: SourceProductName=Aerospace Blockset  SourceProductBaseCode=AE
  Minus2 : Sum
  Minus5 : Sum  Inputs=+-
  Mux3 : Mux  Inputs=2
  Mux4 : Mux  Inputs=2
  Prelookup : PreLookup  BreakpointsData=piece.Nl  BreakpointObject=Nl  ExtrapMethod=Linear  UseLastBreakpoint=on  DiagnosticForOutOfRangeInput=Warning
  Reshape4 : Reshape  OutputDimensionality=Row vector (2-D)
  S_s : sharedschedule/Interpolate Matrix(x)   matrix=piece.K_s  aMode=aMode
      settings: SourceProductName=Aerospace Blockset  SourceProductBaseCode=AE
  Selector : Selector  InputPortWidth=2  IndexOptions=Index vector (dialog)  Indices=[1]  OutputSizes=1
  "kalman " : Subsystem
  steadyHP : sharedschedule/Interpolate Matrix(x)   matrix=piece.steadyHP  aMode=aMode
      settings: SourceProductName=Aerospace Blockset  SourceProductBaseCode=AE
  steadyOutput : sharedschedule/Interpolate Matrix(x)   matrix=piece.steadyOutput  aMode=aMode
      settings: SourceProductName=Aerospace Blockset  SourceProductBaseCode=AE
  steadyState : sharedschedule/Interpolate Matrix(x)   matrix=piece.steadyState  aMode=aMode
      settings: SourceProductName=Aerospace Blockset  SourceProductBaseCode=AE
  steadyinput : sharedschedule/Interpolate Matrix(x)   matrix=piece.steadyInput  aMode=aMode
      settings: SourceProductName=Aerospace Blockset  SourceProductBaseCode=AE
  hp_est : Outport
  y_est : Outport  Port=2
  wires:
  Reshape4/1 -> hp_est/1
  Prelookup/2 -> A/2, S_s/2, K/2, D_k/2, C_k/2, B_k/2, A_k/2, M/2, L/2, steadyHP/2, steadyOutput/2, steadyState/2, steadyinput/2, D/2, C/2, B/2
  Prelookup/1 -> S_s/1, K/1, D_k/1, C_k/1, B_k/1, A_k/1, M/1, L/1, steadyHP/1, steadyOutput/1, steadyState/1, steadyinput/1, D/1, C/1, B/1, A/1
  K/1 -> "kalman "/3(K)
  Selector/1 -> Prelookup/1
  x0/1 -> Mux4/1
  A_k/1 -> "kalman "/1(A)
  "kalman "/1(X_es) -> Demux2/1
  Demux2/1 -> Selector/1
  "kalman "/2(Y_es) -> Minus2/1
  Mux3/1 -> "kalman "/6(Xtrim)
  y/1 -> Minus5/1
  Minus5/1 -> "kalman "/5(Y)
  Demux2/2 -> Reshape4/1
  C_k/1 -> "kalman "/2(C)
  "y_obem "/1 -> Minus2/2, Minus5/2
  Mux4/1 -> "kalman "/4(x0)
  Constant6/1 -> Mux4/2
  steadyHP/1 -> Mux3/2
  Minus2/1 -> y_est/1
  x_obem/1 -> Mux3/1

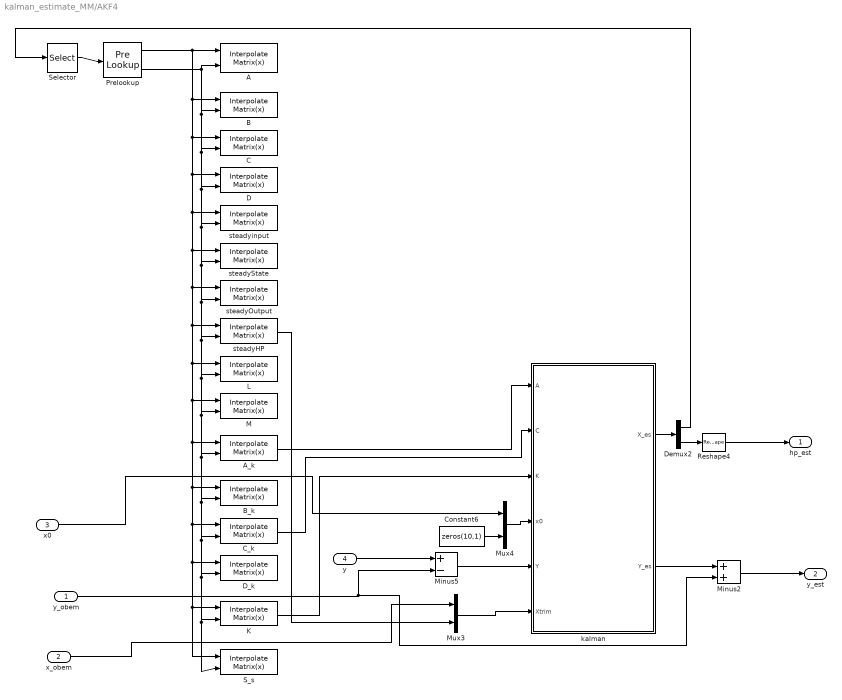
== system kalman_estimate_MM/AKF4 ==
  "y_obem " : Inport
  x_obem : Inport  Port=2
  x0 : Inport  Port=3
  y : Inport  Port=4
  A : sharedschedule/Interpolate Matrix(x)   matrix=piece.A  aMode=aMode
      settings: SourceProductName=Aerospace Blockset  SourceProductBaseCode=AE
  A_k : sharedschedule/Interpolate Matrix(x)   matrix=piece.A_k  aMode=aMode
      settings: SourceProductName=Aerospace Blockset  SourceProductBaseCode=AE
  B : sharedschedule/Interpolate Matrix(x)   matrix=piece.B  aMode=aMode
      settings: SourceProductName=Aerospace Blockset  SourceProductBaseCode=AE
  B_k : sharedschedule/Interpolate Matrix(x)   matrix=piece.B_k  aMode=aMode
      settings: SourceProductName=Aerospace Blockset  SourceProductBaseCode=AE
  C : sharedschedule/Interpolate Matrix(x)   matrix=piece.C  aMode=aMode
      settings: SourceProductName=Aerospace Blockset  SourceProductBaseCode=AE
  C_k : sharedschedule/Interpolate Matrix(x)   matrix=piece.C_k  aMode=aMode
      settings: SourceProductName=Aerospace Blockset  SourceProductBaseCode=AE
  Constant6 : Constant  Value=zeros(10,1)  VectorParams1D=off
  D : sharedschedule/Interpolate Matrix(x)   matrix=piece.D  aMode=aMode
      settings: SourceProductName=Aerospace Blockset  SourceProductBaseCode=AE
  D_k : sharedschedule/Interpolate Matrix(x)   matrix=piece.D_k  aMode=aMode
      settings: SourceProductName=Aerospace Blockset  SourceProductBaseCode=AE
  Demux2 : Demux  Outputs=[2,10]
  K : sharedschedule/Interpolate Matrix(x)   matrix=piece.K  aMode=aMode
      settings: SourceProductName=Aerospace Blockset  SourceProductBaseCode=AE
  L : sharedschedule/Interpolate Matrix(x)   matrix=piece.L  aMode=aMode
      settings: SourceProductName=Aerospace Blockset  SourceProductBaseCode=AE
  M : sharedschedule/Interpolate Matrix(x)   matrix=piece.M  aMode=aMode
      settings: SourceProductName=Aerospace Blockset  SourceProductBaseCode=AE
  Minus2 : Sum
  Minus5 : Sum  Inputs=+-
  Mux3 : Mux  Inputs=2
  Mux4 : Mux  Inputs=2
  Prelookup : PreLookup  BreakpointsData=piece.Nl  BreakpointObject=Nl  ExtrapMethod=Linear  UseLastBreakpoint=on  DiagnosticForOutOfRangeInput=Warning
  Reshape4 : Reshape  OutputDimensionality=Row vector (2-D)
  S_s : sharedschedule/Interpolate Matrix(x)   matrix=piece.K_s  aMode=aMode
      settings: SourceProductName=Aerospace Blockset  SourceProductBaseCode=AE
  Selector : Selector  InputPortWidth=2  IndexOptions=Index vector (dialog)  Indices=[1]  OutputSizes=1
  "kalman " : Subsystem
  steadyHP : sharedschedule/Interpolate Matrix(x)   matrix=piece.steadyHP  aMode=aMode
      settings: SourceProductName=Aerospace Blockset  SourceProductBaseCode=AE
  steadyOutput : sharedschedule/Interpolate Matrix(x)   matrix=piece.steadyOutput  aMode=aMode
      settings: SourceProductName=Aerospace Blockset  SourceProductBaseCode=AE
  steadyState : sharedschedule/Interpolate Matrix(x)   matrix=piece.steadyState  aMode=aMode
      settings: SourceProductName=Aerospace Blockset  SourceProductBaseCode=AE
  steadyinput : sharedschedule/Interpolate Matrix(x)   matrix=piece.steadyInput  aMode=aMode
      settings: SourceProductName=Aerospace Blockset  SourceProductBaseCode=AE
  hp_est : Outport
  y_est : Outport  Port=2
  wires:
  x_obem/1 -> Mux3/1
  Minus2/1 -> y_est/1
  steadyHP/1 -> Mux3/2
  Constant6/1 -> Mux4/2
  Mux4/1 -> "kalman "/4(x0)
  "y_obem "/1 -> Minus5/2, Minus2/2
  C_k/1 -> "kalman "/2(C)
  Demux2/2 -> Reshape4/1
  Minus5/1 -> "kalman "/5(Y)
  y/1 -> Minus5/1
  Mux3/1 -> "kalman "/6(Xtrim)
  "kalman "/2(Y_es) -> Minus2/1
  Demux2/1 -> Selector/1
  "kalman "/1(X_es) -> Demux2/1
  A_k/1 -> "kalman "/1(A)
  x0/1 -> Mux4/1
  Selector/1 -> Prelookup/1
  K/1 -> "kalman "/3(K)
  Prelookup/1 -> A/1, B/1, C/1, D/1, steadyinput/1, steadyState/1, steadyOutput/1, steadyHP/1, L/1, M/1, A_k/1, B_k/1, C_k/1, D_k/1, K/1, S_s/1
  Prelookup/2 -> B/2, C/2, D/2, steadyinput/2, steadyState/2, steadyOutput/2, steadyHP/2, L/2, M/2, A_k/2, B_k/2, C_k/2, D_k/2, K/2, S_s/2, A/2
  Reshape4/1 -> hp_est/1
